simulink model "lab0_3"  (R2021a)
settings: Solver=VariableStepAuto  StartTime=0.0  StopTime=10  RelTol=1e-3
settings Model: Creator=Giancarlo  LastModifiedBy=Giancarlo

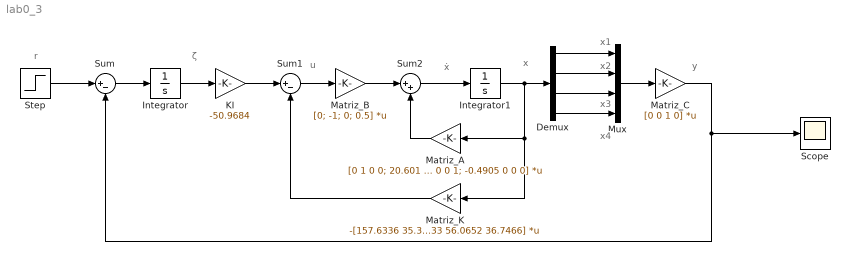
== system lab0_3 ==
  note: x4
  note: x3
  note: x2
  note: x1
  note: ẋ
  note: y
  note: x
  note: u
  note: ζ
  note: r
  Demux : Demux
  Integrator : Integrator
  Integrator1 : Integrator
  KI : Gain  Gain=-50.9684
  Matriz_A : Gain  Gain=[0 1 0 0; 20.601 0 0 0; 0 0 0 1; -0.4905 0 0 0]  Multiplication=Matrix(K*u)
  Matriz_B : Gain  Gain=[0; -1; 0; 0.5]  Multiplication=Matrix(K*u)
  Matriz_C : Gain  Gain=[0 0 1 0]  Multiplication=Matrix(K*u)
  Matriz_K : Gain  Gain=-[157.6336 35.3733 56.0652 36.7466]  Multiplication=Matrix(K*u)
  Mux : Mux
  Scope : Scope
  Step : Step  Before=1  SampleTime=0
  Sum : Sum  Inputs=|+-
  Sum1 : Sum  Inputs=|+-
  Sum2 : Sum  Inputs=|++
  wires:
  Step/1 -> Sum/1
  Sum/1 -> Integrator/1
  Integrator/1 -> KI/1
  KI/1 -> Sum1/1
  Matriz_K/1 -> Sum1/2
  Sum1/1 -> Matriz_B/1
  Matriz_B/1 -> Sum2/1
  Matriz_A/1 -> Sum2/2
  Sum2/1 -> Integrator1/1
  Integrator1/1 -> Matriz_K/1, Matriz_A/1, Demux/1
  Demux/1 -> Mux/1
  Demux/2 -> Mux/2
  Demux/3 -> Mux/3
  Demux/4 -> Mux/4
  Mux/1 -> Matriz_C/1
  Matriz_C/1 -> Sum/2, Scope/1
